simulink model "gravity_precise_model"  (R2018a)
settings: Solver=VariableStepAuto  StartTime=0.0  StopTime=10.0  RelTol=1e-3
undefined symbols (not defined in the file or in its folder): Earth, WGS84
libraries: simulink x2, aerolibasang x2, aerolib6dof2 x1, aerolibanim x1, aerolibadyn x1, aerolibatmos2 x1
settings Model: Creator=annakooperberg  LastModifiedBy=annakooperberg

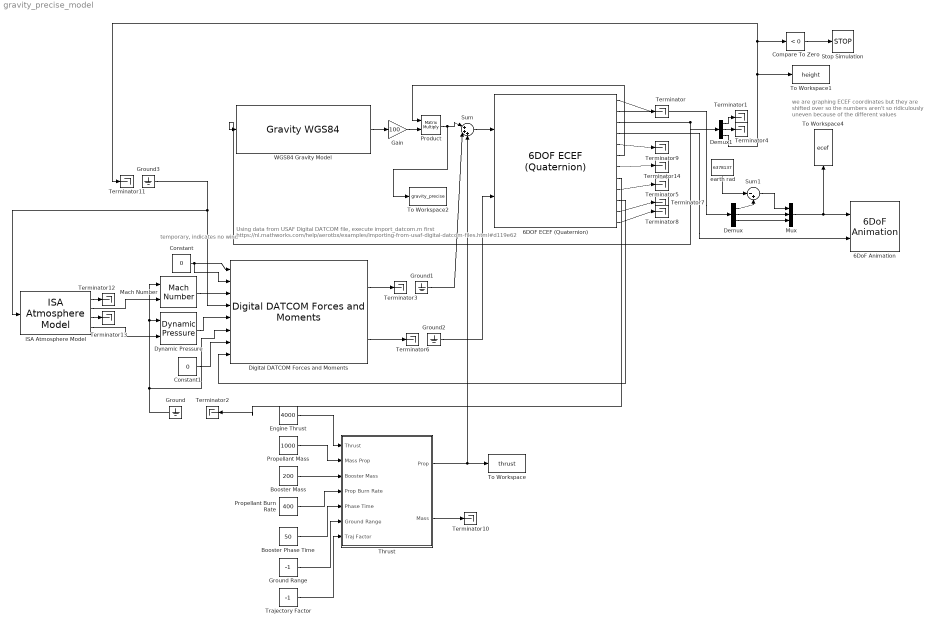
== system gravity_precise_model ==
  note: temporary,
      | indicates no
      | wind
  note: Using data from USAF Digital DATCOM file, execute import_datcom.m first
      | https://nl.mathworks.com/help/aerotbx/examples/importing-from-usaf-digital-datcom-files.html#d119e62
  note: we are graphing ECEF coordinates
      | but they are shifted over so the numbers aren't
      | so ridiculously uneven because of the different
      | values
  6DOF ECEF (Quaternion) : aerolib6dof2/6DOF ECEF (Quaternion)  units=Metric (MKS)  mtype=Fixed  xg_0=[0 0 0]  Vm_0=[0 0 0]  eul_0=[0 pi/4 0]  pm_0=[0 0 0]  mass_0=100  mass_e=0.5  mass_f=2.0  inertia=eye(3)  inertia_e=eye(3)  inertia_f=2*eye(3)  vre_flag=on  abi_flag=off  ptype=Earth (WGS84)  R=6378137  F=1/298.257223563  w_E=7292115e-11  angle_in=Internal  LG0=0
      settings: SourceProductName=Aerospace Blockset  SourceProductBaseCode=AE
  6DoF Animation : aerolibanim/6DoF Animation  u1=[-1000 1000 -1000 1000 -1000 1000]  u2=0.1  u3=1  u4=[4000 0 -5000]  u5=Fixed position  u6=[2000 500 -3150]  u7=10  u8=on
      settings: SourceProductName=Aerospace Blockset
  Booster Mass : Constant  Value=200
  Booster Phase Time : Constant  Value=50
  Compare To Zero : simulink/Logic and Bit Operations/Compare To Zero  relop=<  OutDataTypeStr=boolean
  Constant : Constant  Value=0
  Constant1 : Constant  Value=0
  Demux : Demux  Outputs=3
  Demux1 : Demux  Outputs=3
  Digital DATCOM Forces and Moments : aerolibadyn/Digital DATCOM Forces and Moments  units=Metric (MKS)  dcase=data  fmode=Body  buildno=0  imethod=None - flat  emethod=None - clip  rmethod=Clip to Range  action=None
      settings: SourceProductName=Aerospace Blockset  SourceProductBaseCode=AE
  Dynamic Pressure : aerolibasang/Dynamic Pressure
  Engine Thrust : Constant  Value=4000
  Gain : Gain  Gain=100
  Ground{,1..3} (4 alike) : Ground
  Ground Range : Constant  Value=-1
  ISA Atmosphere Model : aerolibatmos2/ISA Atmosphere Model  custom=off  g=9.80665  gamma=1.4  R=287.0531  L=0.0065  h_trop=11000  h_strat=20000  rho0=1.225  P0=101325  T0=288.15  h0=0
      settings: SourceProductName=Aerospace Blockset
  Mach Number : aerolibasang/Mach Number
      settings: SourceProductName=Aerospace Blockset  SourceProductBaseCode=AE
  Mux : Mux  Inputs=3
  Product : Product  Multiplication=Matrix(*)
  Propellant Burn Rate : Constant  Value=400
  Propellant Mass : Constant  Value=1000
  Stop Simulation : Stop
  Sum : Sum  Inputs=|+++
  Sum1 : Sum  Inputs=|-+
  Terminator{,1..14} (15 alike) : Terminator
  Thrust : Subsystem
  To Workspace : ToWorkspace  VariableName=thrust  SaveFormat=Timeseries  SampleTime=-1
  To Workspace1 : ToWorkspace  VariableName=height  SaveFormat=Timeseries  SampleTime=-1
  To Workspace2 : ToWorkspace  VariableName=gravity_precise  SaveFormat=Timeseries  SampleTime=-1
  To Workspace4 : ToWorkspace  VariableName=ecef  SaveFormat=Timeseries  SampleTime=-1
  Trajectory Factor : Constant  Value=-1
  "WGS84 Gravity Model  " : GravityWGS84
  earth rad : Constant  Value=6378137
  wires:
  Sum/1 -> 6DOF ECEF (Quaternion)/1
  6DOF ECEF (Quaternion)/12 -> Terminator8/1
  Digital DATCOM Forces and Moments/2 -> Terminator6/1
  Demux1/1 -> Terminator1/1
  ISA Atmosphere Model/2 -> Mach Number/2
  Mach Number/1 -> Digital DATCOM Forces and Moments/3
  Compare To Zero/1 -> Stop Simulation/1
  Demux1/2 -> Terminator4/1
  Thrust/2(Mass) -> Terminator10/1
  6DOF ECEF (Quaternion)/8 -> Terminator2/1
  Engine Thrust/1 -> Thrust/1(Thrust)
  Thrust/1(Prop) -> Sum/3, To Workspace/1
  Dynamic Pressure/1 -> Digital DATCOM Forces and Moments/5
  Trajectory Factor/1 -> Thrust/7(Traj Factor)
  Booster Phase Time/1 -> Thrust/5(Phase Time)
  Propellant Mass/1 -> Thrust/2(Mass Prop)
  Digital DATCOM Forces and Moments/1 -> Terminator3/1
  6DOF ECEF (Quaternion)/1 -> Terminator/1
  Constant1/1 -> Digital DATCOM Forces and Moments/7
  Ground Range/1 -> Thrust/6(Ground Range)
  Sum1/1 -> Mux/1
  Demux1/3 -> Terminator11/1, Compare To Zero/1, To Workspace1/1
  6DOF ECEF (Quaternion)/10 -> Digital DATCOM Forces and Moments/8
  Demux/3 -> Mux/3
  6DOF ECEF (Quaternion)/4 -> 6DoF Animation/2
  Demux/2 -> Mux/2
  Constant/1 -> Digital DATCOM Forces and Moments/2, Digital DATCOM Forces and Moments/1
  Mux/1 -> To Workspace4/1, 6DoF Animation/1
  Propellant Burn Rate/1 -> Thrust/4(Prop Burn Rate)
  ISA Atmosphere Model/4 -> Dynamic Pressure/2
  6DOF ECEF (Quaternion)/11 -> Terminator7/1
  6DOF ECEF (Quaternion)/2 -> Demux/1
  Booster Mass/1 -> Thrust/3(Booster Mass)
  6DOF ECEF (Quaternion)/3 -> "WGS84 Gravity Model  "/1, Demux1/1
  earth rad/1 -> Sum1/1
  Demux/1 -> Sum1/2
  Ground/1 -> Mach Number/1, Dynamic Pressure/1, Digital DATCOM Forces and Moments/6
  6DOF ECEF (Quaternion)/9 -> Terminator5/1
  6DOF ECEF (Quaternion)/5 -> Terminator9/1
  Ground2/1 -> 6DOF ECEF (Quaternion)/2
  Ground3/1 -> ISA Atmosphere Model/1, Digital DATCOM Forces and Moments/4
  ISA Atmosphere Model/1 -> Terminator12/1
  ISA Atmosphere Model/3 -> Terminator13/1
  Ground1/1 -> Sum/2
  "WGS84 Gravity Model  "/1 -> Gain/1
  6DOF ECEF (Quaternion)/6 -> Product/1
  6DOF ECEF (Quaternion)/7 -> Terminator14/1
  Gain/1 -> Product/2
  Product/1 -> To Workspace2/1, Sum/1

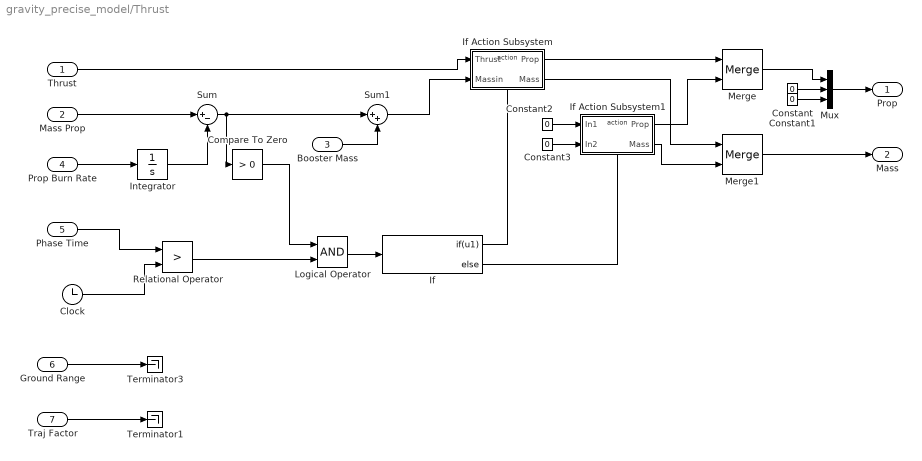
== system gravity_precise_model/Thrust ==
  Thrust : Inport
  Mass Prop : Inport  Port=2
  Booster Mass : Inport  Port=3
  Prop Burn Rate : Inport  Port=4
  Phase Time : Inport  Port=5
  Ground Range : Inport  Port=6
  Traj Factor : Inport  Port=7
  Clock : Clock
  Compare To Zero : simulink/Logic and Bit Operations/Compare To Zero  relop=>  OutDataTypeStr=boolean
  Constant{,1..3} (4 alike) : Constant  Value=0
  If : If  IfExpression=u1
  If Action Subsystem : Subsystem  TreatAsAtomicUnit=on
  If Action Subsystem1 : Subsystem  TreatAsAtomicUnit=on
  Integrator : Integrator
  Logical Operator : Logic  AllPortsSameDT=off  OutDataTypeStr=boolean
  Merge : Merge
  Merge1 : Merge
  Mux : Mux  Inputs=3
  Relational Operator : RelationalOperator  Operator=>  OutDataTypeStr=boolean  RndMeth=Nearest
  Sum : Sum  Inputs=|+-
  Sum1 : Sum  Inputs=|++
  Terminator1 : Terminator
  Terminator3 : Terminator
  Prop : Outport
  Mass : Outport  Port=2
  wires:
  Phase Time/1 -> Relational Operator/1
  If Action Subsystem/1(Prop) -> Merge/1
  Thrust/1 -> If Action Subsystem/1(Thrust)
  Mass Prop/1 -> Sum/1
  If/1 -> If Action Subsystem/Action
  Merge/1 -> Mux/1
  Compare To Zero/1 -> Logical Operator/1
  Clock/1 -> Relational Operator/2
  Relational Operator/1 -> Logical Operator/2
  Prop Burn Rate/1 -> Integrator/1
  If Action Subsystem1/1(Prop) -> Merge/2
  Constant1/1 -> Mux/3
  Mux/1 -> Prop/1
  If/2 -> If Action Subsystem1/Action
  Constant/1 -> Mux/2
  Sum/1 -> Sum1/1, Compare To Zero/1
  Logical Operator/1 -> If/1
  Integrator/1 -> Sum/2
  Sum1/1 -> If Action Subsystem/2(Massin)
  Booster Mass/1 -> Sum1/2
  If Action Subsystem/2(Mass) -> Merge1/1
  If Action Subsystem1/2(Mass) -> Merge1/2
  Merge1/1 -> Mass/1
  Constant3/1 -> If Action Subsystem1/2(In2)
  Constant2/1 -> If Action Subsystem1/1(In1)
  Traj Factor/1 -> Terminator1/1
  Ground Range/1 -> Terminator3/1

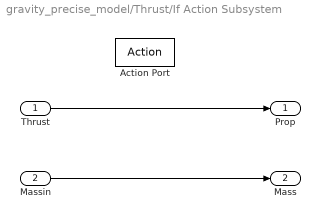
== system gravity_precise_model/Thrust/If Action Subsystem ==
  Thrust : Inport
  Massin : Inport  Port=2
  Action Port : ActionPort  ActionType=then
  Prop : Outport
  Mass : Outport  Port=2
  wires:
  Thrust/1 -> Prop/1
  Massin/1 -> Mass/1

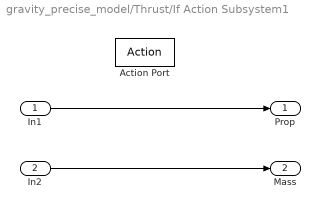
== system gravity_precise_model/Thrust/If Action Subsystem1 ==
  In1 : Inport
  In2 : Inport  Port=2
  Action Port : ActionPort  ActionType=else
  Prop : Outport
  Mass : Outport  Port=2
  wires:
  In1/1 -> Prop/1
  In2/1 -> Mass/1
